simulink model "EXP2_sim"  (R2021b)
settings: Solver=ode1  StartTime=0.0  StopTime=1.0  FixedStep=0.0001  RelTol=1e-3
settings Model: Creator=henri  LastModifiedBy=luanf
settings SolverCC: AlgebraicLoopSolver=TrustRegion
settings DebuggingCC: SFMachineParentedDataDiag=warning
settings SFSimCC: CustomCodeUndefinedFunction=UseInterfaceOnly

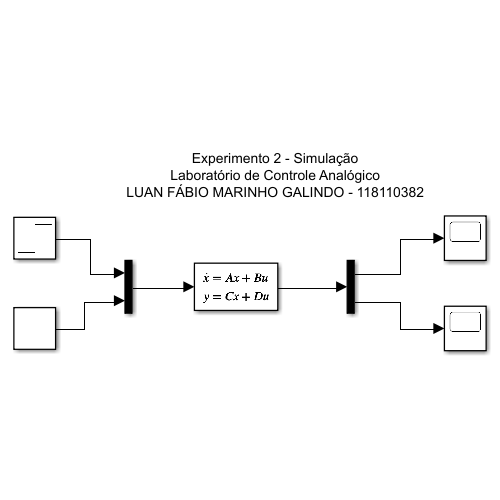
[thumbnail: Simulink's stored preview of the top-level diagram]
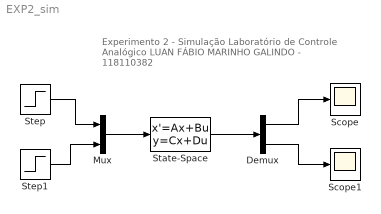
== system EXP2_sim ==
  note: Experimento 2 - Simulação
      | Laboratório de Controle Analógico
      | LUAN FÁBIO MARINHO GALINDO - 118110382
  Demux : Demux  Outputs=2
  Mux : Mux  Inputs=2
  Scope : Scope
  Scope1 : Scope
  State-Space : StateSpace  A=[-33.333333333333336,-4.444444444444445e+02;8,-0.100000000000000]  B=[5.555555555555555e+02,0;0,-10]  C=[1,0;0,1]  D=[0,0;0,0]  InitialCondition=0
  Step : Step  Time=0  SampleTime=0
  Step1 : Step  Time=0  SampleTime=0
  wires:
  Step1/1 -> Mux/2
  Step/1 -> Mux/1
  Mux/1 -> State-Space/1
  State-Space/1 -> Demux/1
  Demux/1 -> Scope/1
  Demux/2 -> Scope1/1
